simulink subsystem "MPC1_nlpsol"  (R2022b)
settings: Solver=VariableStepAuto  StartTime=0.0  StopTime=10.0  RelTol=1e-3
undefined symbols (not defined in the file): param_MPC1, param_traj_data, param_weight_init
settings Model: Creator=emu  LastModifiedBy=emu
settings OptimizationCC: ReuseModelBlockBuffer=on

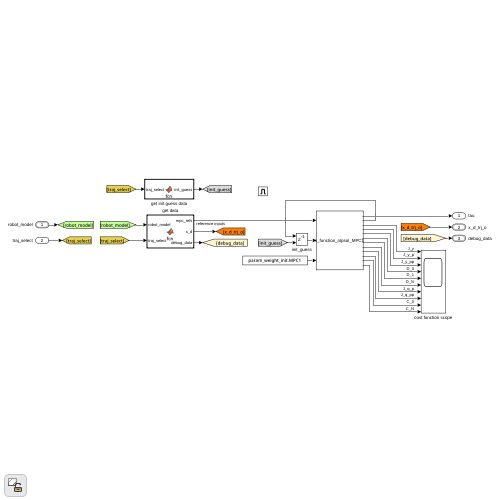
[thumbnail: Simulink's stored preview of the top-level diagram]
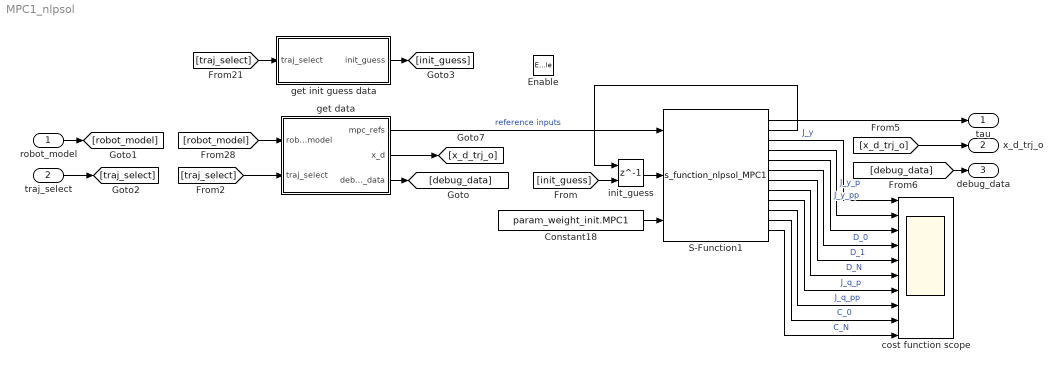
== system MPC1_nlpsol ==
  robot_model : Inport  OutDataTypeStr=Bus: robot_model
  traj_select : Inport  Port=2
  Enable : EnablePort
  Constant18 : Constant  Value=param_weight_init.MPC1  VectorParams1D=off
  S-Function1 : S-Function  FunctionName=s_function_nlpsol_MPC1  Parameters='s_functions/s_functions_2dof/MPC1.casadi', 'MPC1'  SFunctionModules='MPC1'  SFunctionDeploymentMode=off  EnableBusSupport=off
  cost function scope : Scope  NumInputPorts=10
  get data : MATLAB Function  TreatAsAtomicUnit=on
  get init guess data : MATLAB Function  TreatAsAtomicUnit=on
  init_guess : Delay  DelayLength=1  InitialConditionSource=Input port  InitialCondition=1
      settings: InputPortMap=u0,p4
  tau : Outport
  x_d_trj_o : Outport  Port=2  OutDataTypeStr=Bus: x_d
  debug_data : Outport  Port=3  OutDataTypeStr=Bus: debug_data_bus
  wires:
  [traj_select] -> get data/2(traj_select)
  S-Function1/5 -> cost function scope/3  "J_y_pp"
  [debug_data] -> debug_data/1
  robot_model/1 -> [robot_model]
  S-Function1/6 -> cost function scope/4  "D_0"
  [robot_model] -> get data/1(robot_model)
  get data/1(mpc_refs) -> S-Function1/1  "reference inputs"
  S-Function1/1 -> tau/1
  S-Function1/9 -> cost function scope/7  "J_q_p"
  Constant18/1 -> S-Function1/3
  traj_select/1 -> [traj_select]
  init_guess/1 -> S-Function1/2
  [x_d_trj_o] -> x_d_trj_o/1
  S-Function1/4 -> cost function scope/2  "J_y_p"
  S-Function1/10 -> cost function scope/8  "J_q_pp"
  S-Function1/2 -> init_guess/1
  [init_guess] -> init_guess/2
  S-Function1/11 -> cost function scope/9  "C_0"
  S-Function1/3 -> cost function scope/1  "J_y"
  S-Function1/7 -> cost function scope/5  "D_1"
  S-Function1/12 -> cost function scope/10  "C_N"
  get init guess data/1(init_guess) -> [init_guess]
  get data/3(debug_data) -> [debug_data]
  [traj_select] -> get init guess data/1(traj_select)
  get data/2(x_d) -> [x_d_trj_o]
  S-Function1/8 -> cost function scope/6  "D_N"

== matlab function MPC1_nlpsol/get data ==
  settings: updateMethod=DISCRETE  sampleTime=param_global.Ta
  data: mpc_refs output; robot_model input Bus: robot_model; param_MPC1 parameter; x_d output Bus: x_d; debug_data output Bus: debug_data_bus; param_traj_data parameter; traj_select input
function [mpc_refs, x_d, debug_data] = fcn(robot_model, param_MPC1, param_traj_data, traj_select)
persistent cnt;

if(isempty(cnt))
    cnt = 1;
end

param_MPC = param_MPC1;
N         = param_MPC.N;
N_step    = param_MPC.N_step;

% Parameters
q    = robot_model.q;      % generalized coordinates
q_p  = robot_model.q_p;  % time derivative of generalized coordinates
q_pp = robot_model.q_pp;
H    = robot_model.H;
J    = robot_model.J;
J_p  = robot_model.J_p;

% Current Pose of Endeffector
p = H(1:2,4);
p_p = J(1:2,1:2)*q_p;
p_pp = J(1:2,1:2)*q_pp + J_p(1:2,1:2)*q_p;

R = H(1:3,1:3);

% desired Orientation as Rotationmatrix
q_e = rotation2quaternion(R);

% Error of Position (translation) and first time derivative
q_err = quat_mult(q_e, quat_inv(param_traj_data.q_d(1:4, cnt, traj_select)));

x_k = [q;q_p];

% Assemble vector of recieved output measurements
p_d_traj    = param_traj_data.p_d(   1:3, cnt : N_step : cnt + (N  )*N_step, traj_select);
p_d_p_traj  = param_traj_data.p_d_p( 1:3, cnt : N_step : cnt + (N  )*N_step, traj_select);
p_d_pp_traj = param_traj_data.p_d_pp(1:3, cnt : N_step : cnt + (N-1)*N_step, traj_select);

y_ref    = p_d_traj(   1:2, 1 + (1:N  ) ); %       y1,   y2,   ... yN
y_ref_p  = p_d_p_traj( 1:2, 1 + (1:N  ) ); %       y1p,  y2p,  ... yNp
y_ref_pp = p_d_pp_traj(1:2, 1 + (0:N-1) ); % y0pp, y1pp, y2pp, ... yN-1pp

cnt = cnt+1;

%% Reference out

mpc_refs = [x_k(:); y_ref(:); y_ref_p(:); y_ref_pp(:)];

%% TRAJECTORY OUT
x_d.p_d       = p_d_traj(1:3,1);    %y0
x_d.p_d_p     = p_d_p_traj(1:3,1);  %y0p
x_d.p_d_pp    = p_d_pp_traj(1:3,1); %y0pp
x_d.q_d       = [0; 0; 0; 0];
x_d.omega_d   = [0; 0; 0];
x_d.omega_d_p = [0; 0; 0];

%% DEBUG
debug_data.p    = p(1:2);
debug_data.p_p  = p_p(1:2);
debug_data.p_pp = p_pp(1:2);
debug_data.rot_x_err = q_err(2);
debug_data.rot_y_err = q_err(3);
debug_data.rot_z_err = q_err(4);

== matlab function MPC1_nlpsol/get init guess data ==
  data: traj_select input; param_MPC1_init_guess parameter; init_guess output
function init_guess  = fcn(traj_select, param_MPC1_init_guess)

init_guess = param_MPC1_init_guess.init_guess(traj_select,:);
